simulink library "bcm"  (R2021b)
settings: Solver=VariableStepAuto  StartTime=0.0  StopTime=10.0  RelTol=1e-3
undefined symbols (not defined in the file or in its folder): ENUM_ANTITHEFT_ALARM, ENUM_ANTITHEFT_ARM, ENUM_ANTITHEFT_DISARM, ENUM_ANTITHEFT_WAIT, ENUM_GEARPOSNTOCAN_P, ENUM_PDKEYRAWLULOCK_INUNLOCK, ENUM_PDKEYRAWPS_INPS, ENUM_POWERSTA_READY, ENUM_POWERSTA_STANDBY, FALSE, KBCM_ALMBrightnessDark_enum, KBCM_AmbBlue_enum, KBCM_AmbBreathT_K, KBCM_AmbBreathTOut_K, KBCM_AmbGreen_enum, KBCM_AmbLightUser_enum, KBCM_AmbPreset_enum, KBCM_AmbRed_enum, KBCM_Antitheft_enum_ovrdflg, KBCM_Antitheft_enum_ovrdval, KBCM_APMDoorCtrlSta_flg_ovrdflg, KBCM_APMDoorCtrlSta_flg_ovrdval, KBCM_DelayTSW_flg, KBCM_DiagFLTC_mA, KBCM_DiagFMHT_s, KBCM_DiagFRTC_mA, KBCM_DiagRLTC_mA, KBCM_DiagRRTC_mA, KBCM_DrAPMRetryTimes_cnt, KBCM_DrOpenWdwOT_s, KBCM_DrOpenWdwReady_s, KBCM_ESSOffT_ms, KBCM_ESSOnT_ms, KBCM_IVIRstHoldT_ms, KBCM_IVIRstTriggerT_ms, KBCM_ONDelayT_ms, KBCM_ReDetectT_K, KBCM_RmLampKeep_min, KBCM_RmLpKeyInT_s, KBCM_RmLpKeyMissT_s, KBCM_SlpDebounceTime_s, KBCM_SPTGDetectT_sec, KBCM_SPTGLeave_flg, KBCM_SPTGLeftBound_cm, KBCM_SPTGLeftBoundOut_cm, KBCM_SPTGLowerBound_cm, KBCM_SPTGLowerBoundOut_cm, KBCM_SPTGRightBound_cm, KBCM_SPTGRightBoundOut_cm, KBCM_SPTGTOut_K, KBCM_SPTGUpperBound_cm, KBCM_SPTGUpperBoundOut_cm, KBCM_SPTGWaitDKC_sec, KBCM_USSDis_cm, KBCM_USSFilterT_K, KBCM_WaitAPMPwr_K, KBCM_WdwManualDetT_s, MIN2SEC, TRUE, XX2KXX
libraries: simulink x41, $bdroot x3, hcu_lib x2
(part 6 of 6)

== stateflow chart bcm/BCM/BCM/IVI Reset/Chart ==
  state sRelease
    en:
    VBCM_IVIRST_flg = FALSE;
  state sPress
  state sIVI_RESET_SEND
    en:
    VBCM_IVIRST_flg = TRUE;
  state sSTOP
    en:
    VBCM_IVIRST_flg = FALSE;
  (default) -> sRelease
  sRelease -> sPress : [VINP_SWCmodeSta_flg]
  sPress -> sRelease [order 1] : [!VINP_SWCmodeSta_flg]
  sPress -> sIVI_RESET_SEND [order 2] : [after(KBCM_IVIRstTriggerT_ms,tick)]
  sIVI_RESET_SEND -> sSTOP : [after(KBCM_IVIRstHoldT_ms,tick)]
  sSTOP -> sRelease : [!VINP_SWCmodeSta_flg]
  data: KBCM_IVIRstHoldT_ms input; KBCM_IVIRstTriggerT_ms input; VINP_SWCmodeSta_flg input; VBCM_IVIRST_flg output; FALSE parameter; TRUE parameter

== stateflow chart bcm/BCM/BCM/PTG/Chart ==
  state NoDetected
    en:
    VBCM_SPTGDet_flg=0;
    VBCM_APSOpenPTG_flg=0;
  state Alarm
    en:
    VBCM_SPTGDet_flg=1;
  state WaitForDKC
  state DoorOpen
    en:
    VBCM_SPTGDet_flg=0;
    VBCM_APSOpenPTG_flg=1;
  state WaitforLeave
    en:
    VBCM_APSOpenPTG_flg=0;
    VBCM_SPTGDet_flg=0;
    state OutRange
    state InRange
    (default) -> InRange
    InRange -> OutRange : [(PASDRMR>=100 || PASDRML>=100) && (!TailgateSW)]
    OutRange -> InRange [order 1] : [(PASDRMR<100 && PASDRML<100) || TailgateSW]
  (junction 109) -> NoDetected [order 1] : [KBCM_DelayTSW_flg==0]{VBCM_u8DetectWaitT_s=0;}
  Alarm -> (junction 109) [order 1] : [hasChangedTo(KeyDetectedOut,0)&&KBCM_SPTGLeave_flg==1]
  (junction 109) -> (junction 70) [order 2]
  (junction 70) -> NoDetected : {VBCM_u8DetectWaitT_s=100;}
  (junction 128) -> Alarm
  WaitForDKC -> (junction 128) [order 1] : [PDKeyAreaPTG==1]
  NoDetected -> NoDetected [order 2] : [VBCM_u8DetectWaitT_s>0]{VBCM_u8DetectWaitT_s=VBCM_u8DetectWaitT_s-1;}
  Alarm -> WaitforLeave [order 2] : [ShiftGearPosn!=0||....
      | VehSpeed>0||....
      | PwrSta==5||....
      | TailgateSW!=0||....
      | IVI_PTG_USSta_SW!=0||....
      | PDKeyAreaPTG!=1]
  Alarm -> WaitforLeave [order 3] : [DKCKeyPress]
  Alarm -> DoorOpen [order 4] : [after(KBCM_SPTGDetectT_sec*100,tick)]
  NoDetected -> WaitForDKC [order 1] : [hasChangedTo(KeyDetected,1)&&VBCM_u8DetectWaitT_s==0....
      | &&....
      | (ShiftGearPosn==0&&....
      | VehSpeed<=0&&....
      | PwrSta!=5&&....
      | TailgateSW==0&&....
      | IVI_PTG_USSta_SW==0)]
  DoorOpen -> WaitforLeave : [after(40,tick)]
  (default) -> WaitforLeave
  (junction 136) -> NoDetected [order 1] : [KBCM_DelayTSW_flg==0]{VBCM_u8DetectWaitT_s=0;}
  WaitForDKC -> (junction 136) [order 2] : [hasChangedTo(KeyDetectedOut,0)&&....
      | KBCM_SPTGLeave_flg==1]
  (junction 136) -> (junction 138) [order 2]
  (junction 138) -> NoDetected : {VBCM_u8DetectWaitT_s=100;}
  WaitForDKC -> WaitforLeave [order 3] : [after(KBCM_SPTGWaitDKC_sec*100,tick)]
  OutRange -> NoDetected [order 2] : after(KBCM_ReDetectT_K,tick)
  data: KBCM_DelayTSW_flg input; KeyDetected input; PASDRMR input; PASDRML input; PDKeyAreaPTG input; PwrSta input; KeyDetectedOut input; TailgateSW input; VehSpeed input; DKCKeyPress input; ShiftGearPosn input; IVI_PTG_USSta_SW input; VBCM_APSOpenPTG_flg output; VBCM_SPTGDet_flg output; VBCM_u8DetectWaitT_s local uint8 =0; KBCM_ReDetectT_K input =1; KBCM_SPTGDetectT_sec input; KBCM_SPTGLeave_flg input; KBCM_SPTGWaitDKC_sec input

== stateflow chart bcm/BCM/BCM/APM_Door/DoorAPM/window ==
  state Normal
    state DoorClose
      state NoResponse
      state PwrOpenReq
        en:CtrlCmd = 126;
      state WinClose
        en:CtrlCmd = 0;
        ex:CtrlCmd = 127;
      state StandBy
      (default) -> (junction 123)
      (junction 123) -> (junction 124) [order 1] : [ Val_Wdw_Opened > 10....
          | ||....
          | Val_Wdw_Opened <= 0 ]
      (junction 123) -> (junction 58) [order 2]
      (junction 124) -> Normal.DoorClose.NoResponse
      (junction 58) -> (junction 56) [order 1] : [!CANMsgValidGWZoneDR1....
          | ||....
          | !CANMsgValidGWZoneFR1]
      (junction 56) -> Normal.DoorClose.NoResponse [order 2]
      (junction 58) -> WinClose [order 2]
      (junction 56) -> Normal.DoorClose.PwrOpenReq [order 1] : [DrAPMRetryCnt<KBCM_DrAPMRetryTimes_cnt]
      (junction 130) -> Normal.DoorClose.NoResponse
      Normal.DoorClose.PwrOpenReq -> WinClose [order 1] : [CANMsgValidGWZoneDR1....
          | &&....
          | CANMsgValidGWZoneFR1]
      WinClose -> Normal.DoorClose.StandBy : [Val_Wdw_Opened <= 0 || ...
          | after(DrOpenWdwOT_K,tick)]
      Normal.DoorClose.PwrOpenReq -> (junction 99) [order 2]
      (junction 99) -> Normal.DoorClose.StandBy : [after(WaitAPMPwr_K,tick)]
          | {CtrlCmd=127;
          | DrAPMRetryCnt=DrAPMRetryCnt+1;}
      Normal.DoorClose.StandBy -> (junction 130) [order 1] : [hasChanged(Val_Wdw_Opened)]
    state DoorOpen
      state NoResponse
      state WinOpen
        en:CtrlCmd = 6;
        ex:CtrlCmd = 127;
      state PwrOpenReq
        en:CtrlCmd = 126;
      state StandBy
      (default) -> (junction 48)
      (junction 48) -> (junction 120) [order 1]
      (junction 48) -> (junction 51) [order 2] : [!CANMsgValidGWZoneDR1....
          | ||....
          | !CANMsgValidGWZoneFR1]
      (junction 51) -> Normal.DoorOpen.NoResponse [order 2]
      (junction 120) -> Normal.DoorOpen.StandBy : [ Val_Wdw_Opened > 0 ]
      (junction 48) -> WinOpen [order 3]
      (junction 51) -> Normal.DoorOpen.PwrOpenReq [order 1] : [DrAPMRetryCnt<KBCM_DrAPMRetryTimes_cnt]
      Normal.DoorOpen.PwrOpenReq -> WinOpen [order 1] : [CANMsgValidGWZoneDR1....
          | &&....
          | CANMsgValidGWZoneFR1]
      Normal.DoorOpen.PwrOpenReq -> (junction 102) [order 2]
      WinOpen -> Normal.DoorOpen.StandBy : [Val_Wdw_Opened >= 6 || ...
          | after(DrOpenWdwOT_K,tick)]
      (junction 102) -> Normal.DoorOpen.StandBy : [after(WaitAPMPwr_K,tick)]
          | {CtrlCmd=127;
          | DrAPMRetryCnt=DrAPMRetryCnt+1;}
    state Reverse
    (default) -> DoorClose
    (junction 8) -> DoorClose [order 1] : [!DoorSW]
    (junction 8) -> DoorOpen [order 2]
    Reverse -> (junction 8) : [CtrlCmd_Ready]
    (junction 21) -> Reverse [order 2]
    DoorClose -> (junction 21) : [DoorSW]
        | {DrAPMRetryCnt=0;}
    (junction 21) -> DoorOpen [order 1] : [CtrlCmd_Ready]
    (junction 29) -> (junction 21) [order 2]
    (junction 29) -> DoorClose [order 1] : [CtrlCmd_Ready]
    DoorOpen -> (junction 29) : [!DoorSW]
        | {DrAPMRetryCnt=0;}
    (junction 94) -> (junction 29)
    Normal.DoorClose.StandBy -> (junction 94) [order 2] : [ Val_Wdw_Opened <= 10 && Val_Wdw_Opened > 0 ]
    Normal.DoorOpen.StandBy -> (junction 94) [order 2] : [ Val_Wdw_Opened <= 0 ]
  state ManualOpen
    en:
    CtrlCmd = 127;
  state IVICmdSend
    en:
    CtrlCmd = ControlCommand_Buf;
  state CommandRst
    en:
    CtrlCmd=127;
  (default) -> ManualOpen
  ManualOpen -> (junction 65) [order 2]
  Normal -> (junction 65) [order 1]
  (junction 65) -> (junction 66) : [hasChangedFrom(ControlCommand, 127)]
      | {ControlCommand_Buf = ControlCommand;}
  (junction 66) -> (junction 79) [order 2]
  (junction 79) -> IVICmdSend
  (junction 66) -> CommandRst [order 1] : [!CtrlCmd_Ready]
  CommandRst -> IVICmdSend : [CtrlCmd_Ready]
  IVICmdSend -> ManualOpen : [after(12,tick)]
  Normal -> ManualOpen [order 2] : [!APMDoorControlSta]
  ManualOpen -> Normal.DoorClose.StandBy [order 1] : [APMDoorControlSta]
      | {DrAPMRetryCnt=0;}
  Normal.DoorOpen.StandBy -> ManualOpen [order 1] : [( hasChanged(Val_Wdw_Opened) && ( Val_Wdw_Opened>=10 ) ) && after(KBCM_WdwManualDetT_K,tick)]
  data: DoorSW input boolean; Val_Wdw_Opened input uint8; WaitAPMPwr_K input uint8; APMDoorControlSta input; CtrlCmd_Ready input; ControlCommand input; DrOpenWdwOT_K input uint8; CtrlCmd output uint8; ControlCommand_Buf local uint8; KBCM_WdwManualDetT_K input; CANMsgValidGWZoneDR1 input boolean; CANMsgValidGWZoneFR1 input boolean; KBCM_DrAPMRetryTimes_cnt input; DrAPMRetryCnt local uint8 =0
